simulink model "differential"  (R2017a)
settings: Solver=VariableStepAuto  StartTime=0.0  StopTime=1.4  MaxStep=1e-4  RelTol=1e-3
libraries: powerlib x11, dspstat3 x6, simulink_extras x3
settings Model: Creator=Waqas  LastModifiedBy=ikon

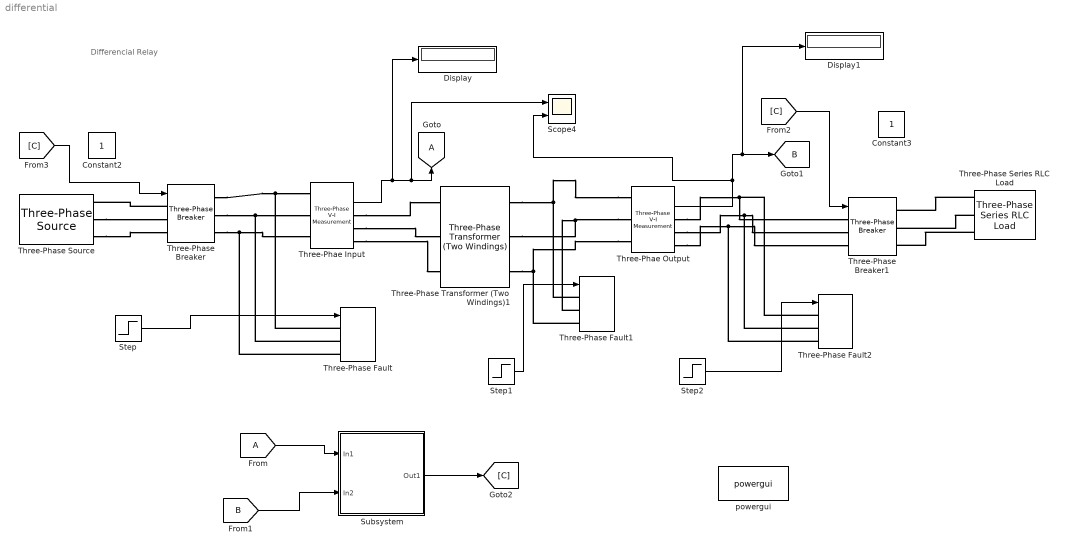
== system differential ==
  note: Differencial Relay
  Constant2 : Constant
  Constant3 : Constant
  Display : Display
  Display1 : Display
  Scope4 : Scope  NumInputPorts=2
  Step : Step  Time=4  SampleTime=0
  Step1 : Step  Time=5  SampleTime=0
  Step2 : Step  SampleTime=0
  Subsystem : Subsystem
  Three-Phae Input : powerlib/Measurements/Three-Phase V-I Measurement  VoltageMeasurement=phase-to-ground  SetLabelV=off  LabelV=Vabc  Vpu=off  VpuLL=off  CurrentMeasurement=yes  SetLabelI=off  LabelI=Iabc  Ipu=off  Pbase=100e6  Vbase=500e3  OutputType=Complex  PhasorSimulation=off  PSBequivalent=0
  Three-Phae Output : powerlib/Measurements/Three-Phase V-I Measurement  VoltageMeasurement=phase-to-ground  SetLabelV=off  LabelV=Vabc  Vpu=off  VpuLL=off  CurrentMeasurement=yes  SetLabelI=off  LabelI=Iabc  Ipu=off  Pbase=100e6  Vbase=500e3  OutputType=Complex  PhasorSimulation=off  PSBequivalent=0
  Three-Phase Series RLC Load : powerlib/Elements/Three-Phase Series RLC Load  LConnTagsString=A|B|C  Configuration=Y (grounded)  NominalVoltage=1000  Vabc=[1e3 1e3 1e3]  Vabcp=[1e3 1e3 1e3]  NominalFrequency=60  UnbalancedPower=off  ActivePower=10e3  InductivePower=100  CapacitivePower=100  Pabc=[10e3 9e3 11e3]  QLabc=[100 90 110]  QCabc=[100 90 110]  Pabcp=[10e3 9e3 11e3]  QLabcp=[100 90 110]  QCabcp=[100 90 110]  Measurements=None  LoadType=constant Z
  Three-Phase Transformer (Two Windings)1 : powerlib/Elements/Three-Phase Transformer (Two Windings)  Winding1Connection=Yg  Winding2Connection=Yg  CoreType=Three single-phase transformers  SetSaturation=off  Hysteresis=off  DataFile='hysteresis'  SetInitialFlux=off  Measurements=None  UNITS=pu  NominalPower=[ 250e6 , 60 ]  Winding1=[ 735e3 , 0.002 , 0.08 ]  Winding2=[ 735e3 , 0.002 , 0.08 ]  Rm=500  Lm=500  L0=0.5  Saturation=[ 0,0 ; 0.0024,1.2 ; 1.0,1.52 ]  InitialFluxes=[ 0.8 , -0.8 , 0.7 ]  MoreParameters=off  BreakLoop=off  DataType=off  TransfoNumber=1
  Three-Phase Breaker : powerlib/Elements/Three-Phase Breaker  InitialState=closed  SwitchA=on  SwitchB=off  SwitchC=on  SwitchTimes="[1/60  5/60]"  External=on  BreakerResistance=0.01  SnubberResistance=1e6  SnubberCapacitance=inf  Measurements=None
  Three-Phase Breaker1 : powerlib/Elements/Three-Phase Breaker  InitialState=closed  SwitchA=on  SwitchB=on  SwitchC=on  SwitchTimes="[1/60  5/60]"  External=on  BreakerResistance=0.01  SnubberResistance=1e6  SnubberCapacitance=inf  Measurements=None
  Three-Phase Fault : powerlib/Elements/Three-Phase Fault  InitialStates=0  FaultA=on  FaultB=on  FaultC=on  GroundFault=on  SwitchTimes="[1/60  5/60]"  External=on  SwitchStatus=NaN  FaultResistance=0.001  GroundResistance=0.01  SnubberResistance=1e6  SnubberCapacitance=inf  Measurements=None
  Three-Phase Fault1 : powerlib/Elements/Three-Phase Fault  InitialStates=0  FaultA=on  FaultB=on  FaultC=on  GroundFault=on  SwitchTimes="[1/60  5/60]"  External=on  SwitchStatus=NaN  FaultResistance=0.001  GroundResistance=0.01  SnubberResistance=1e6  SnubberCapacitance=inf  Measurements=None
  Three-Phase Fault2 : powerlib/Elements/Three-Phase Fault  InitialStates=0  FaultA=on  FaultB=on  FaultC=on  GroundFault=on  SwitchTimes="[1/60  5/60]"  External=on  SwitchStatus=NaN  FaultResistance=0.001  GroundResistance=0.01  SnubberResistance=1e6  SnubberCapacitance=inf  Measurements=None
  Three-Phase Source : powerlib/Electrical Sources/Three-Phase Source  InternalConnection=Yg  VoltagePhases=off  Voltage=735e3  PhaseAngle=0  Voltage_phases=[25e3 25e3 25e3]/sqrt(3)  PhaseAngles_phases=[0 -120 +120]  Frequency=60  NonIdealSource=on  SpecifyImpedance=off  Resistance=0.8929  Inductance=16.58e-3  ShortCircuitLevel=100e6  BaseVoltage=25e3  XRratio=7  BusType=swing  Pref=10e3  Qref=0  Prefabc=[10e3, 10e3, 10e3]  Qrefabc=[0, 0, 0]  Qmin=-inf  Qmax=inf
  powergui : powerlib/powergui  Priority=1  SimulationMode=Continuous  SampleTime=50e-6  frequency=60  Iterations=50  frequencyindice=60  Pbase=100e6  ErrMax=1e-4  UnitsV=kV  UnitsW=MW  buscounter=0  FunctionMessages=off  echomessages=off  EnableUseOfTLC=off  CurrentSourceSwitches=off  DisableSnubberDevices=off  DisableRonSwitches=off  DisableVfSwitches=off  DisplayEquations=off  SolverType=Tustin/Backward Euler (TBE)  Interpol=off  ExternalGateDelay=off  methode=off  Ts=100  x0status=blocks  SPID=on  SwTol=0  HookPort=off  RestoreLinks=warning  ResistiveCurrentMeasurement=off  Frange=[0:2:500]  Ylog=off  Xlog=on  ShowGrid=off  save=off  variable=ZData  structure=0  ZoomFFT=off  StartTime=0.0  cycles=1  DisplayStyle=1  fundamental=60  FreqAxis=off  MaxFrequency=1000  frequencyindicesteady=1  RmsSteady=1  display=off
  tag scope: A=global, B=global
  wires:
  Step/1 -> Three-Phase Fault/1
  Step1/1 -> Three-Phase Fault1/1
  Step2/1 -> Three-Phase Fault2/1
  Three-Phae Output/2 -> Scope4/2, Display1/1, [B]
  Three-Phae Input/2 -> Display/1, Scope4/1, [A]
  [C] -> Three-Phase Breaker/1
  [C] -> Three-Phase Breaker1/1
  [B] -> Subsystem/2(In2)
  [A] -> Subsystem/1(In1)
  Subsystem/1(Out1) -> [C]
  connections:
  Three-Phase Breaker/LConn1 -- Three-Phase Source/RConn1
  Three-Phase Source/RConn2 -- Three-Phase Breaker/LConn2
  Three-Phase Source/RConn3 -- Three-Phase Breaker/LConn3
  Three-Phase Breaker/RConn1 -- Three-Phase Fault/LConn1 -- Three-Phae Input/LConn1
  Three-Phase Breaker/RConn2 -- Three-Phase Fault/LConn2 -- Three-Phae Input/LConn2
  Three-Phase Breaker/RConn3 -- Three-Phase Fault/LConn3 -- Three-Phae Input/LConn3
  Three-Phae Input/RConn1 -- Three-Phase Transformer (Two Windings)1/LConn1
  Three-Phae Input/RConn2 -- Three-Phase Transformer (Two Windings)1/LConn2
  Three-Phae Input/RConn3 -- Three-Phase Transformer (Two Windings)1/LConn3
  Three-Phae Output/LConn1 -- Three-Phase Transformer (Two Windings)1/RConn1 -- Three-Phase Fault1/LConn1
  Three-Phae Output/LConn2 -- Three-Phase Transformer (Two Windings)1/RConn2 -- Three-Phase Fault1/LConn2
  Three-Phae Output/LConn3 -- Three-Phase Transformer (Two Windings)1/RConn3 -- Three-Phase Fault1/LConn3
  Three-Phae Output/RConn1 -- Three-Phase Fault2/LConn1 -- Three-Phase Breaker1/LConn1
  Three-Phae Output/RConn2 -- Three-Phase Fault2/LConn2 -- Three-Phase Breaker1/LConn2
  Three-Phae Output/RConn3 -- Three-Phase Fault2/LConn3 -- Three-Phase Breaker1/LConn3
  Three-Phase Series RLC Load/LConn1 -- Three-Phase Breaker1/RConn1
  Three-Phase Series RLC Load/LConn2 -- Three-Phase Breaker1/RConn2
  Three-Phase Series RLC Load/LConn3 -- Three-Phase Breaker1/RConn3

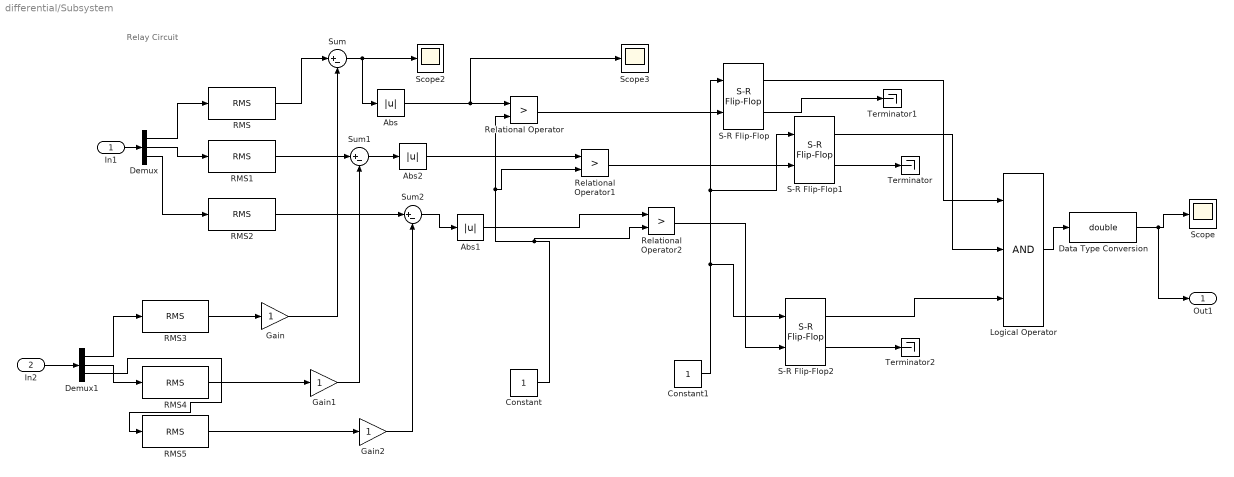
== system differential/Subsystem ==
  note: Relay Circuit
  In1 : Inport
  In2 : Inport  Port=2
  Abs : Abs
  Abs1 : Abs
  Abs2 : Abs
  Constant : Constant
  Constant1 : Constant  OutDataTypeStr=boolean
  Data Type Conversion : DataTypeConversion  OutDataTypeStr=double
  Demux : Demux  Outputs=3
  Demux1 : Demux  Outputs=3
  Gain : Gain
  Gain1 : Gain
  Gain2 : Gain
  Logical Operator : Logic  Inputs=3  AllPortsSameDT=off  OutDataTypeStr=boolean
  RMS{,1..5} (6 alike) : dspstat3/RMS  run=off  directionMode=Each column  dimension=1  InputProcessing=Columns as channels (frame based)  reset_popup=None
  Relational Operator : RelationalOperator  Operator=>  OutDataTypeStr=boolean  RndMeth=Simplest
  Relational Operator1 : RelationalOperator  Operator=>  OutDataTypeStr=boolean  RndMeth=Simplest
  Relational Operator2 : RelationalOperator  Operator=>  OutDataTypeStr=boolean  RndMeth=Simplest
  S-R Flip-Flop : simulink_extras/Flip Flops/S-R Flip-Flop  initial_condition=0
  S-R Flip-Flop1 : simulink_extras/Flip Flops/S-R Flip-Flop  initial_condition=0
  S-R Flip-Flop2 : simulink_extras/Flip Flops/S-R Flip-Flop  initial_condition=0
  Scope : Scope
  Scope2 : Scope
  Scope3 : Scope
  Sum : Sum  Inputs=|+-
  Sum1 : Sum  Inputs=|+-
  Sum2 : Sum  Inputs=|+-
  Terminator : Terminator
  Terminator1 : Terminator
  Terminator2 : Terminator
  Out1 : Outport
  wires:
  Demux1/1 -> RMS3/1
  Constant1/1 -> S-R Flip-Flop2/1, S-R Flip-Flop1/1, S-R Flip-Flop/1
  RMS5/1 -> Gain2/1
  Gain/1 -> Sum/2
  Data Type Conversion/1 -> Out1/1, Scope/1
  Abs1/1 -> Relational Operator2/1
  RMS4/1 -> Gain1/1
  S-R Flip-Flop/1 -> Logical Operator/1
  S-R Flip-Flop1/1 -> Logical Operator/2
  Demux1/2 -> RMS4/1
  S-R Flip-Flop2/2 -> Terminator2/1
  Demux/3 -> RMS2/1
  S-R Flip-Flop2/1 -> Logical Operator/3
  Logical Operator/1 -> Data Type Conversion/1
  Demux/1 -> RMS/1
  Relational Operator/1 -> S-R Flip-Flop/2
  Demux1/3 -> RMS5/1
  RMS3/1 -> Gain/1
  Relational Operator1/1 -> S-R Flip-Flop1/2
  RMS2/1 -> Sum2/1
  Sum1/1 -> Abs2/1
  Constant/1 -> Relational Operator2/2, Relational Operator1/2, Relational Operator/2
  Relational Operator2/1 -> S-R Flip-Flop2/2
  Abs/1 -> Scope3/1, Relational Operator/1
  Demux/2 -> RMS1/1
  Sum2/1 -> Abs1/1
  S-R Flip-Flop1/2 -> Terminator/1
  Sum/1 -> Scope2/1, Abs/1
  Gain2/1 -> Sum2/2
  RMS1/1 -> Sum1/1
  RMS/1 -> Sum/1
  Gain1/1 -> Sum1/2
  Abs2/1 -> Relational Operator1/1
  S-R Flip-Flop/2 -> Terminator1/1
  In1/1 -> Demux/1
  In2/1 -> Demux1/1
